simulink model "test_02"  (R2017b)
settings: Solver=VariableStepAuto  StartTime=0.0  StopTime=10.0  RelTol=1e-3
settings Model: Creator=flosch  LastModifiedBy=flosch
settings ConfigComp: CovScope=ReferencedModels  CovIncludeTopModel=off

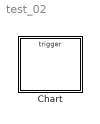
== system test_02 ==
  Chart : Stateflow chart  TreatAsAtomicUnit=on

== stateflow chart test_02/Chart ==
  state L1_A
    state L2_A
    state L2_B
    (default) -> L2_A
    L2_A -> L2_B : Event_B
  state L1_B
    state L2_C
    state L2_D
      state L3_A
      state L3_B
      (default) -> L3_A
      L3_A -> L3_B : Event_C
    (default) -> L2_C
    L2_C -> L2_D : Event_B
  note: cyc = 14
  (default) -> L1_A
  L1_A -> L1_B : Event_A
  L1_B -> L1_A : Event_A
  events: Event_A input RISING_EDGE_EVENT; Event_B input RISING_EDGE_EVENT; Event_C input RISING_EDGE_EVENT
